simulink model "uz_flux_estimator"  (R2024b)
settings: Solver=FixedStepAuto  StartTime=0.0  StopTime=2  RelTol=1e-3
values from neighbouring files (symbols this model uses):
  HPdenum = Hochdenum{1,1}    [parameterierung_Flussschaetzer.m]
  HPnum = Hochnum{1,1}    [parameterierung_Flussschaetzer.m]
  Ls = 1.626e-3    (= 0.001626)    [parameterierung_Flussschaetzer.m]
  p = 1    [parameterierung_Flussschaetzer.m]
  Rs = 7.3    [parameterierung_Flussschaetzer.m]
  THP = 1/(2*pi*fHP)    (= 0.0345989006722)    [parameterierung_Flussschaetzer.m]
  Ts = 1/(2e4)    (= 5e-05)    [parameterierung_Flussschaetzer.m]
undefined symbols (not defined in the file or in its folder): DiscIntNeverNeededParam, dspblkCoreblockFVToolHelper, gcbh, TTP
libraries: eeGeneralControl x1
settings Model: Creator=ELSYS  LastModifiedBy=ELSYS
settings OptimizationCC: OptimizeBlockIOStorage=off  OptimizeDataStoreBuffers=off  BusAssignmentInplaceUpdate=off
settings DebuggingCC: SFUnexpectedBacktrackingDiag=warning  SFNoUnconditionalDefaultTransitionDiag=warning
settings RTWCC: GenerateReport=on  BuildConfiguration=Debug  LaunchReport=on
settings CodeAppCC: ForceParamTrailComments=on  MATLABSourceComments=on  EnableCustomComments=on
settings GRTTargetCC: CombineSignalStateStructs=on  CodeInterfacePackaging=Reusable function  SupportVariableSizeSignals=on  GenerateAllocFcn=on  MultiInstanceErrorCode=Warning

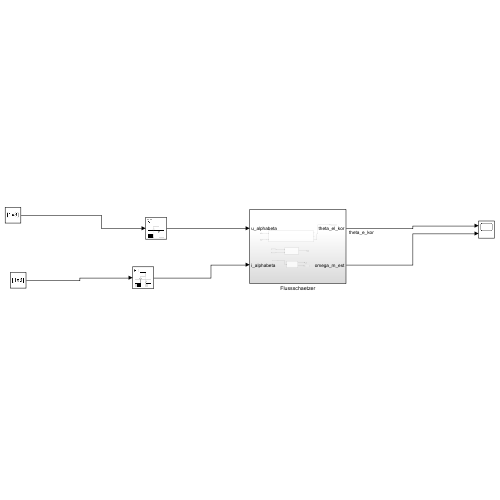
[thumbnail: Simulink's stored preview of the top-level diagram]
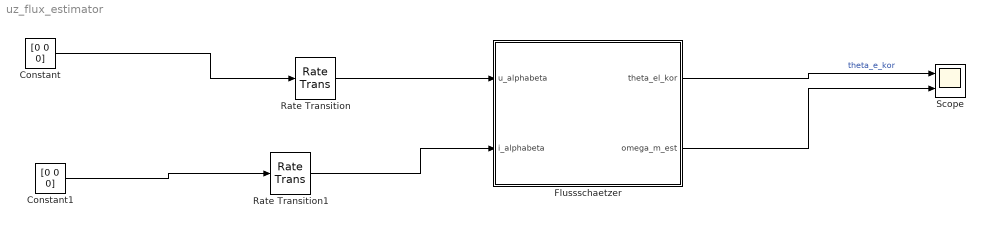
== system uz_flux_estimator ==
  Constant : Constant  Value=[0 0 0]  OutDataTypeStr=single
  Constant1 : Constant  Value=[0 0 0]  OutDataTypeStr=single
  Flussschaetzer : Subsystem
  Rate Transition : RateTransition  OutPortSampleTime=1/20e3
  Rate Transition1 : RateTransition  OutPortSampleTime=1/20e3
  Scope : Scope  NumInputPorts=2
  wires:
  Flussschaetzer/2(omega_m_est) -> Scope/2
  Flussschaetzer/1(theta_el_kor) -> Scope/1  "theta_e_kor"
  Constant1/1 -> Rate Transition1/1
  Constant/1 -> Rate Transition/1
  Rate Transition/1 -> Flussschaetzer/1(u_alphabeta)
  Rate Transition1/1 -> Flussschaetzer/2(i_alphabeta)

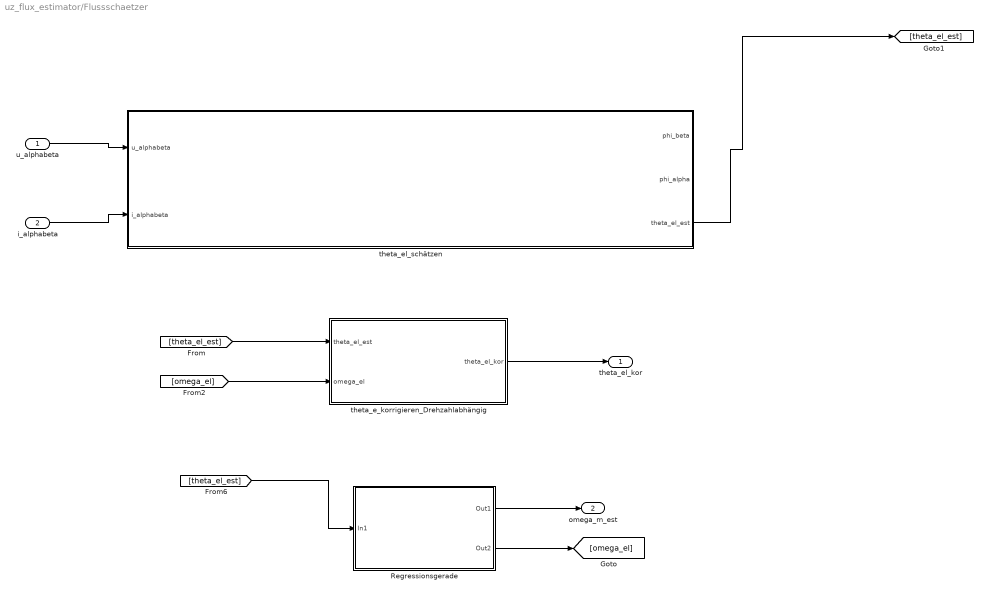
== system uz_flux_estimator/Flussschaetzer ==
  u_alphabeta : Inport
  i_alphabeta : Inport  Port=2
  Regressionsgerade : Subsystem
  theta_e_korrigieren_Drehzahlabhängig : Subsystem
  theta_el_schätzen : Subsystem
  theta_el_kor : Outport
  omega_m_est : Outport  Port=2
  wires:
  theta_e_korrigieren_Drehzahlabhängig/1(theta_el_kor) -> theta_el_kor/1
  [theta_el_est] -> theta_e_korrigieren_Drehzahlabhängig/1(theta_el_est)
  theta_el_schätzen/3(theta_el_est) -> [theta_el_est]
  u_alphabeta/1 -> theta_el_schätzen/1(u_alphabeta)
  i_alphabeta/1 -> theta_el_schätzen/2(i_alphabeta)
  [omega_el] -> theta_e_korrigieren_Drehzahlabhängig/2(omega_el)
  [theta_el_est] -> Regressionsgerade/1(In1)
  Regressionsgerade/1(Out1) -> omega_m_est/1
  Regressionsgerade/2(Out2) -> [omega_el]

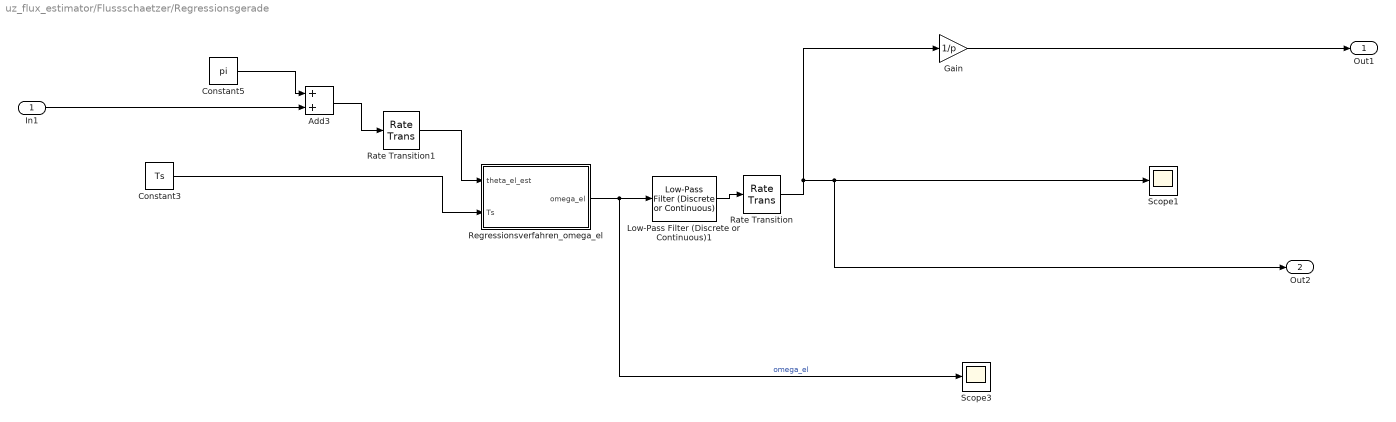
== system uz_flux_estimator/Flussschaetzer/Regressionsgerade ==
  In1 : Inport
  Add3 : Sum
  Constant3 : Constant  Value=Ts
  Constant5 : Constant  Value=pi
  Gain : Gain  Gain=1/p
  Low-Pass Filter (Discrete or Continuous)1 : eeGeneralControl/Low-Pass Filter (Discrete or Continuous)  K=1  T=TTP  B=inf  A=-inf  init_option=Inherited from block input  x0=0  Ts=Ts
  Rate Transition : RateTransition  OutPortSampleTime=Ts
  Rate Transition1 : RateTransition  OutPortSampleTime=Ts
  Regressionsverfahren_omega_el : MATLAB Function  TreatAsAtomicUnit=on
  Scope1 : Scope
  Scope3 : Scope
  Out1 : Outport
  Out2 : Outport  Port=2
  wires:
  Constant5/1 -> Add3/1
  Low-Pass Filter (Discrete or Continuous)1/1 -> Rate Transition/1
  Constant3/1 -> Regressionsverfahren_omega_el/2(Ts)
  Regressionsverfahren_omega_el/1(omega_el) -> Low-Pass Filter (Discrete or Continuous)1/1, Scope3/1  "omega_el"
  Rate Transition/1 -> Out2/1, Scope1/1, Gain/1
  Add3/1 -> Rate Transition1/1
  Rate Transition1/1 -> Regressionsverfahren_omega_el/1(theta_el_est)
  In1/1 -> Add3/2
  Gain/1 -> Out1/1

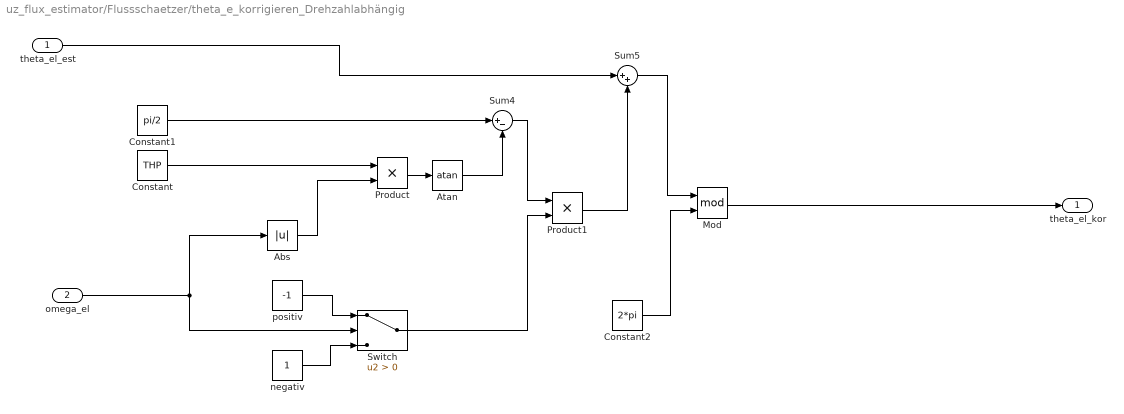
== system uz_flux_estimator/Flussschaetzer/theta_e_korrigieren_Drehzahlabhängig ==
  theta_el_est : Inport
  omega_el : Inport  Port=2
  Abs : Abs  SaturateOnIntegerOverflow=off
  Atan : Trigonometry  Operator=atan
  Constant : Constant  Value=THP
  Constant1 : Constant  Value=pi/2
  Constant2 : Constant  Value=2*pi
  Mod : Math  Operator=mod
  Product : Product
  Product1 : Product
  Sum4 : Sum  Inputs=|+-
  Sum5 : Sum  Inputs=|++
  Switch : Switch  Criteria=u2 > Threshold  SaturateOnIntegerOverflow=off  InputSameDT=off
  negativ : Constant
  positiv : Constant  Value=-1
  theta_el_kor : Outport
  wires:
  theta_el_est/1 -> Sum5/1
  omega_el/1 -> Abs/1, Switch/2
  negativ/1 -> Switch/3
  Product/1 -> Atan/1
  Constant1/1 -> Sum4/1
  Mod/1 -> theta_el_kor/1
  Product1/1 -> Sum5/2
  Constant/1 -> Product/1
  Sum4/1 -> Product1/1
  Abs/1 -> Product/2
  Atan/1 -> Sum4/2
  Sum5/1 -> Mod/1
  positiv/1 -> Switch/1
  Switch/1 -> Product1/2
  Constant2/1 -> Mod/2

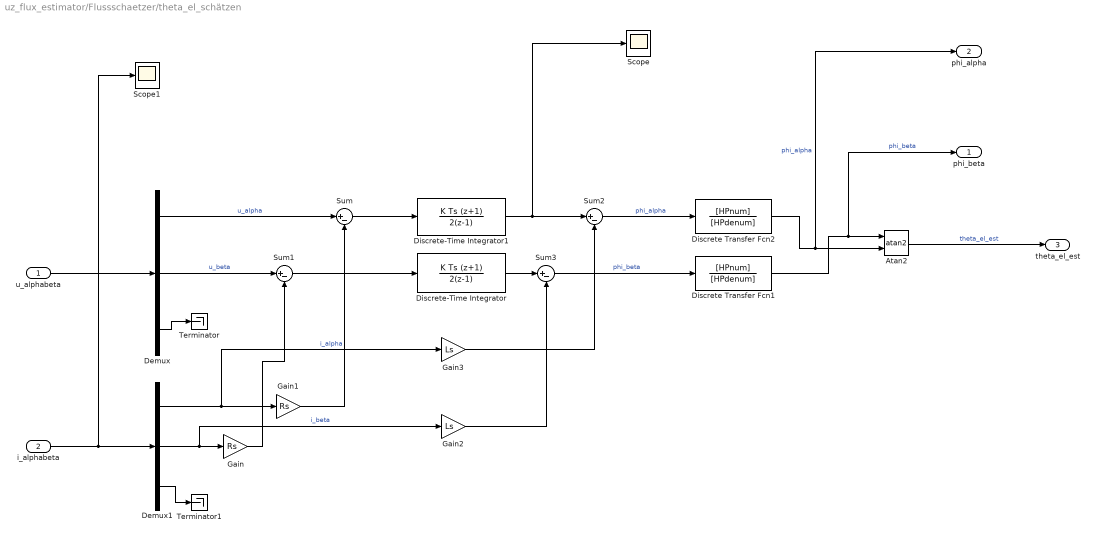
== system uz_flux_estimator/Flussschaetzer/theta_el_schätzen ==
  u_alphabeta : Inport
  i_alphabeta : Inport  Port=2
  Atan2 : Trigonometry  Operator=atan2
  Demux : Demux  Outputs=3
  Demux1 : Demux  Outputs=3
  Discrete Transfer Fcn1 : DiscreteTransferFcn  LoadFcn=dspblkCoreblockFVToolHelper(gcbh,'load');  Numerator=[HPnum]  Denominator=[HPdenum]  InitialStates=1
      settings: CopyFcn=dspblkCoreblockFVToolHelper(gcbh,'copy');  DeleteFcn=dspblkCoreblockFVToolHelper(gcbh,'close');  ModelCloseFcn=dspblkCoreblockFVToolHelper(gcbh,'close');  PreSaveFcn=dspblkCoreblockFVToolHelper(gcbh,'presave');  PostSaveFcn=dspblkCoreblockFVToolHelper(gcbh,'postsave');  CloseFcn=dspblkCoreblockFVToolHelper(gcbh,'close');
  Discrete Transfer Fcn2 : DiscreteTransferFcn  LoadFcn=dspblkCoreblockFVToolHelper(gcbh,'load');  Numerator=[HPnum]  Denominator=[HPdenum]  InitialStates=1
      settings: CopyFcn=dspblkCoreblockFVToolHelper(gcbh,'copy');  DeleteFcn=dspblkCoreblockFVToolHelper(gcbh,'close');  ModelCloseFcn=dspblkCoreblockFVToolHelper(gcbh,'close');  PreSaveFcn=dspblkCoreblockFVToolHelper(gcbh,'presave');  PostSaveFcn=dspblkCoreblockFVToolHelper(gcbh,'postsave');  CloseFcn=dspblkCoreblockFVToolHelper(gcbh,'close');
  Discrete-Time Integrator : DiscreteIntegrator  IntegratorMethod=Integration: Trapezoidal  InitialCondition=1  SampleTime=Ts  ICPrevOutput=DiscIntNeverNeededParam  ICPrevScaledInput=DiscIntNeverNeededParam
  Discrete-Time Integrator1 : DiscreteIntegrator  IntegratorMethod=Integration: Trapezoidal  InitialCondition=1  SampleTime=Ts  ICPrevOutput=DiscIntNeverNeededParam  ICPrevScaledInput=DiscIntNeverNeededParam
  Gain : Gain  Gain=Rs
  Gain1 : Gain  Gain=Rs
  Gain2 : Gain  Gain=Ls
  Gain3 : Gain  Gain=Ls
  Scope : Scope
  Scope1 : Scope
  Sum{,1..3} (4 alike) : Sum  Inputs=|+-
  Terminator : Terminator
  Terminator1 : Terminator
  phi_beta : Outport
  phi_alpha : Outport  Port=2
  theta_el_est : Outport  Port=3
  wires:
  i_alphabeta/1 -> Scope1/1, Demux1/1
  u_alphabeta/1 -> Demux/1
  Gain/1 -> Sum1/2
  Discrete Transfer Fcn1/1 -> Atan2/1, phi_beta/1  "phi_beta"
  Sum2/1 -> Discrete Transfer Fcn2/1  "phi_alpha"
  Discrete-Time Integrator1/1 -> Scope/1, Sum2/1
  Gain1/1 -> Sum/2
  Demux/3 -> Terminator/1
  Gain2/1 -> Sum3/2
  Discrete-Time Integrator/1 -> Sum3/1
  Demux1/3 -> Terminator1/1
  Atan2/1 -> theta_el_est/1  "theta_el_est"
  Demux/2 -> Sum1/1  "u_beta"
  Sum3/1 -> Discrete Transfer Fcn1/1  "phi_beta"
  Gain3/1 -> Sum2/2
  Sum/1 -> Discrete-Time Integrator1/1
  Discrete Transfer Fcn2/1 -> Atan2/2, phi_alpha/1  "phi_alpha"
  Demux/1 -> Sum/1  "u_alpha"
  Demux1/1 -> Gain3/1, Gain1/1  "i_alpha"
  Sum1/1 -> Discrete-Time Integrator/1
  Demux1/2 -> Gain2/1, Gain/1  "i_beta"

== matlab function uz_flux_estimator/Flussschaetzer/Regressionsgerade/Regressionsverfahren_omega_el ==
  data: theta_el_est input; omega_el output; Ts input
function omega_el = fcn(theta_el_est,Ts)


Windowsize = 10;

persistent omega_el_array;
if isempty(omega_el_array)
        omega_el_array = zeros(1, Windowsize); % Initialisierung des Buffers
end

persistent theta_values;
if isempty(theta_values)
        theta_values = zeros(1, Windowsize); % Initialisierung des Buffers
end

% if abs(theta_el_est - mean(theta_values)) >= pi
% 
% theta_values = [theta_values(2:end), mean(theta_values)];
% else 
    theta_values = [theta_values(2:end), theta_el_est];
% end

persistent time_values;
if isempty(time_values)
        time_values = zeros(1, Windowsize); % Initialisierung des Buffers
end
for i = 1: Windowsize
       time_values(1, i) = 1*Ts*i;
end 

% if abs(omega_el_est) <= omega_el_lower1
% omega_el_array = [omega_el_array(2:end), omega_el_est];
% else



time_mean = mean(time_values);
theta_mean = mean(theta_values);
% numerator = sum((time_values - time_mean) .* (theta_values - theta_mean));
% denumerator = sum((time_values - time_mean).^2);
numerator = sum((time_values - time_mean) .* (theta_values - theta_mean));
denumerator = sum((time_values - time_mean).^2);

omega_el_new = numerator / denumerator;

% omega_el = numerator / denumerator;
% end


%if abs((30/pi)*omega_el) <= (omega_el_lower1 - 0.4*omega_el_lower1)

%if abs(omega_el_new - omega_el) >= 50
%    omega_el_array = [omega_el_array(2:end), omega_el];

%else
%    omega_el_array = [omega_el_array(2:end), omega_el_new];
%end
%else 
if abs(omega_el_new - mean(omega_el_array)) >= 50
    omega_el_array = [omega_el_array(2:end), mean(omega_el_array)];

else
    omega_el_array = [omega_el_array(2:end), omega_el_new];
end

%end
omega_el = mean(omega_el_array);
